simulink model "ControlBlockDiagram"  (R2016a)
settings: Solver=VariableStepAuto  StartTime=0.0  StopTime=10.0  RelTol=1e-3
settings Model: Creator=zf1005  LastModifiedBy=zf1005

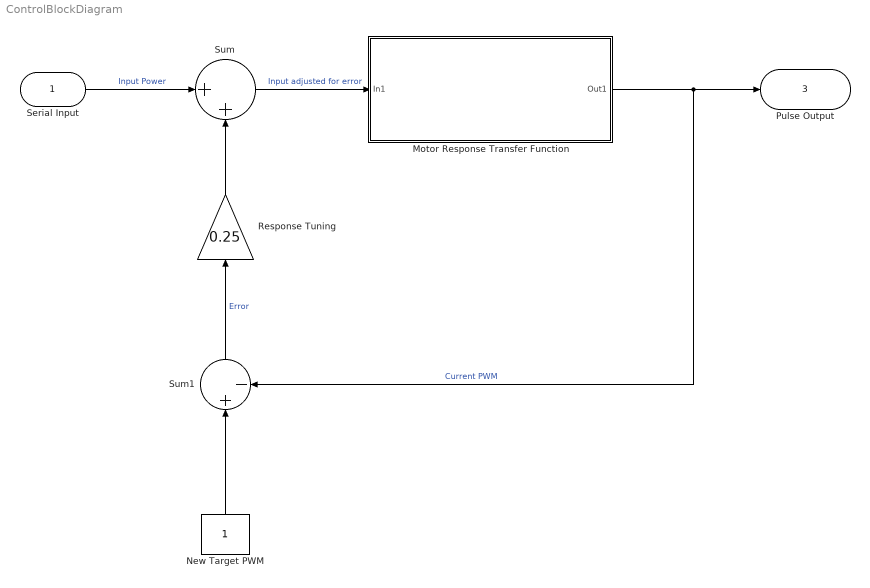
== system ControlBlockDiagram ==
  Serial Input : Inport
  Motor Response Transfer Function : Subsystem
  New Target PWM : Constant
  Response Tuning : Gain  Gain=0.25
  Sum : Sum  Inputs=|++
  Sum1 : Sum  Inputs=|+-
  Pulse Output : Outport  Port=3
  wires:
  Sum/1 -> Motor Response Transfer Function/1(In1)  "Input adjusted for error"
  Motor Response Transfer Function/1(Out1) -> Sum1/2, Pulse Output/1  "Current PWM"
  New Target PWM/1 -> Sum1/1
  Sum1/1 -> Response Tuning/1  "Error"
  Serial Input/1 -> Sum/1  "Input Power"
  Response Tuning/1 -> Sum/2

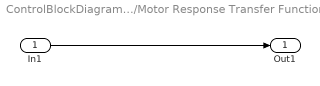
== system ControlBlockDiagram/Motor Response Transfer Function ==
  In1 : Inport
  Out1 : Outport
  wires:
  In1/1 -> Out1/1
